simulink model "damping_model"  (R2024a)
settings: Solver=VariableStepAuto  StartTime=0.0  StopTime=10.0  MaxStep=0.01  RelTol=1e-3
settings Model: Creator=Abbas  LastModifiedBy=Abbas

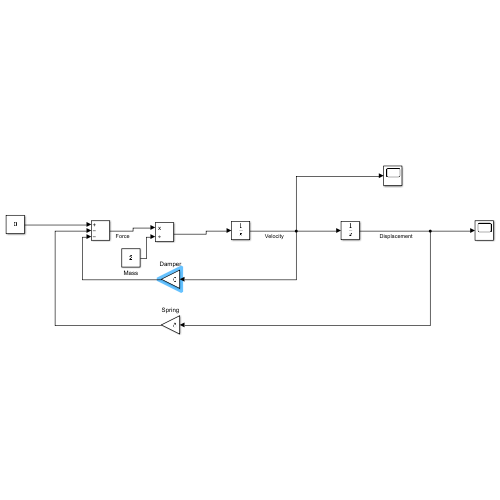
[thumbnail: Simulink's stored preview of the top-level diagram]
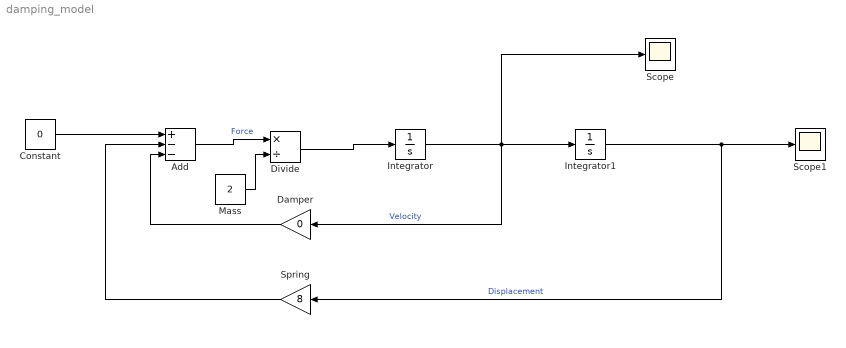
== system damping_model ==
  Add : Sum  Inputs=+--
  Constant : Constant  Value=0
  Damper : Gain  Gain=0
  Divide : Product  Inputs=*/
  Integrator : Integrator  InitialCondition=10
  Integrator1 : Integrator  InitialCondition=0.1
  Mass : Constant  Value=2
  Scope : Scope
  Scope1 : Scope
  Spring : Gain  Gain=8
  wires:
  Integrator/1 -> Scope/1, Damper/1, Integrator1/1  "Velocity"
  Integrator1/1 -> Spring/1, Scope1/1  "Displacement"
  Spring/1 -> Add/2
  Damper/1 -> Add/3
  Constant/1 -> Add/1
  Divide/1 -> Integrator/1
  Add/1 -> Divide/1  "Force"
  Mass/1 -> Divide/2
